simulink model "BMS_EstimateSOC_COM_Harness_MIL"  (R2022b)
settings: configuration reference "BMS_Sw_CodeGenConfig" (kept outside this file)
model workspace: external: MAT-File H:\0\New MAAM\10 - MBD\Battary Management System\SWE.3 CDD\DataTypes\Data_Script.mat (data not in the file)
undefined symbols (not defined in the file): Ion, Lithium
libraries: spsIdealSwitchLib x3, spsBatteryLib x1, spsParallelRLCBranchLib x1, spspowerguiLib x1
settings Model: DataDictionary=BMS_Arch_DD.sldd  Creator=MAAM  LastModifiedBy=MAAM
settings ConfigSetRef: SourceName=BMS_Sw_CodeGenConfig

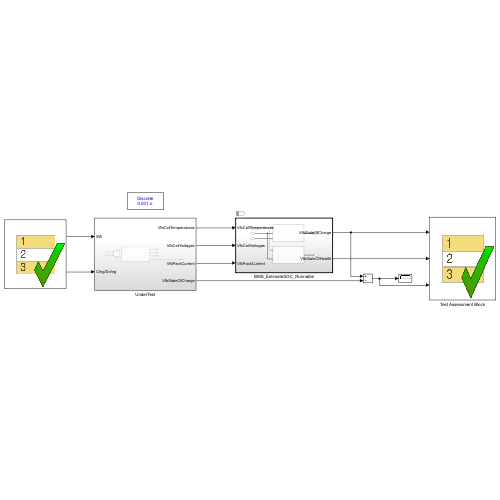
[thumbnail: Simulink's stored preview of the top-level diagram]
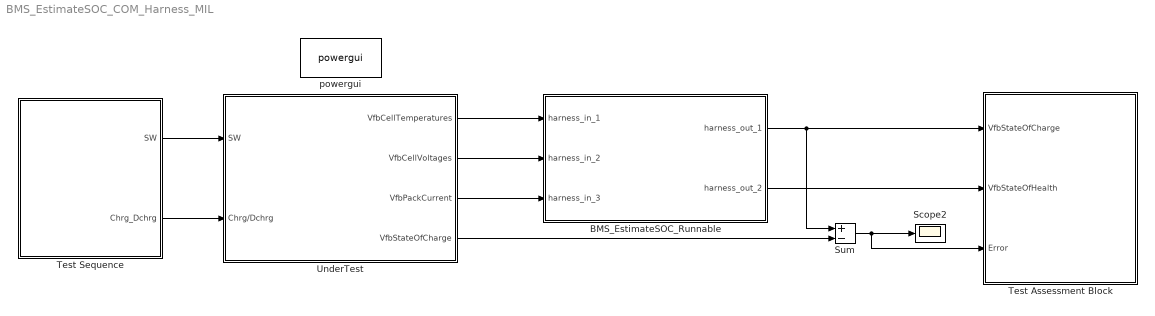
== system BMS_EstimateSOC_COM_Harness_MIL ==
  BMS_EstimateSOC_Runnable : Subsystem  Tag=__SL_testing_harness_stub_  Priority=3
  Scope2 : Scope
  Sum : Sum  Inputs=+-
  Test Assessment Block : Test Sequence  Tag=__SLT_ASMT__  TreatAsAtomicUnit=on
  Test Sequence : Test Sequence  TreatAsAtomicUnit=on
  UnderTest : Subsystem
  powergui : spspowerguiLib/powergui  Priority=1  SimulationMode=Discrete  SampleTime=1e-3  frequency=60  Iterations=50  frequencyindice=0  Pbase=100e6  ErrMax=1e-4  UnitsV=kV  UnitsW=MW  buscounter=0  FunctionMessages=off  echomessages=off  EnableUseOfTLC=off  CurrentSourceSwitches=off  DisableSnubberDevices=off  DisableRonSwitches=off  DisableVfSwitches=off  DisplayEquations=off  AutomaticDiscreteSolvers=off  SolverType=Tustin/Backward Euler (TBE)  Interpol=off  ExternalGateDelay=off  methode=off  Ts=100  x0status=blocks  SPID=on  SwTol=0  HookPort=off  NonlinearTolerance=1e-4  nMaxIteration=100  ContinueOnMaxIteration=off  RestoreLinks=warning  ResistiveCurrentMeasurement=off  Frange=[0:2:500]  Ylog=off  Xlog=on  ShowGrid=off  save=off  variable=ZData  structure=0  ZoomFFT=off  StartTime=0.0  cycles=1  DisplayStyle=1  fundamental=60  FreqAxis=off  MaxFrequency=1000  frequencyindicesteady=1  RmsSteady=1  display=off
  wires:
  BMS_EstimateSOC_Runnable/1(harness_out_1) -> Sum/1, Test Assessment Block/1(VfbStateOfCharge)
  BMS_EstimateSOC_Runnable/2(harness_out_2) -> Test Assessment Block/2(VfbStateOfHealth)
  Sum/1 -> Scope2/1, Test Assessment Block/3(Error)
  Test Sequence/1(SW) -> UnderTest/1(SW)
  Test Sequence/2(Chrg_Dchrg) -> UnderTest/2(Chrg/Dchrg)
  UnderTest/1(VfbCellTemperatures) -> BMS_EstimateSOC_Runnable/1(harness_in_1)
  UnderTest/2(VfbCellVoltages) -> BMS_EstimateSOC_Runnable/2(harness_in_2)
  UnderTest/3(VfbPackCurrent) -> BMS_EstimateSOC_Runnable/3(harness_in_3)
  UnderTest/4(VfbStateOfCharge) -> Sum/2

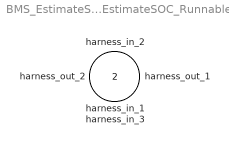
== system BMS_EstimateSOC_COM_Harness_MIL/BMS_EstimateSOC_Runnable ==
  harness_in_1 : Inport
  harness_in_2 : Inport  Port=2
  harness_in_3 : Inport  Port=3
  harness_out_1 : Outport
  harness_out_2 : Outport  Port=2

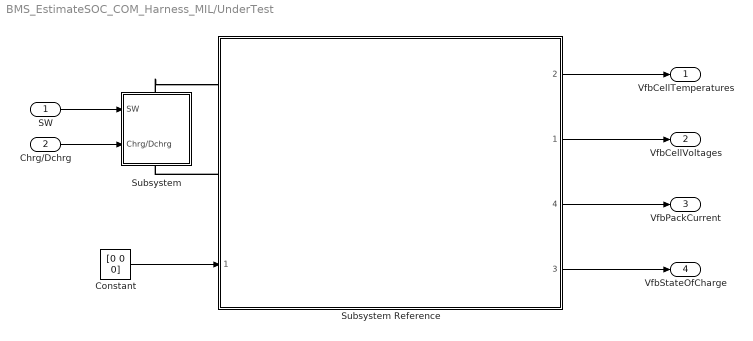
== system BMS_EstimateSOC_COM_Harness_MIL/UnderTest ==
  SW : Inport
  Chrg/Dchrg : Inport  Port=2
  Constant : Constant  Value=[0 0 0]
  Subsystem : Subsystem
      settings: PortSchema="{\"entries\":[{\"content\":{\"sides\":[{\"content\":{\"connectorIds\":[\"LConn1\"]},\"type\":\"ConnectorPlacement.EquallySpacedRectSide\",\"uuid\":\"a461fc5f-bdec-4de1-a769-19a6913359cb\"},{\"content\":{\"connectorIds\":[\"RConn1\"],\"side\":\"RIGHT\"},\"type\":\"ConnectorPlacement.EquallySpacedRectSide\",\"uuid\":\"53dfe770-afde-41f9-b1fd-6523bad3a9ef\"},{\"content\":{\"connectorIds\":[],\"side\":\"TOP\"},\"type\":\"ConnectorPlacement.EquallySpacedRectSide\",\"uuid\":\"157c2878-8b7f-49af-a18e-5ca91668c703\"},{\"content\":{\"connectorIds\":[\"In1\",\"In2\"],\"side\":\"BOTTOM\"},\"type\":\"ConnectorPlacement.EquallySpacedRectSide\",\"uuid\":\"a113e167-ab7e-4584-b97c-54a0a3809f54\"}]},\"type\":\"ConnectorPlacement.EquallySpacedConnector\",\"uuid\":\"fefc71e0-0cbe-4397-b099-f68d58411951\"}],\"packageUris\":[\"http://schema.mathworks.com/mf0/Connector/R2020b\"],\"version\":\"1.0\"}"
  Subsystem Reference : Subsystem  ReferencedSubsystem=Batter_Pack_Sim
      settings: PortSchema="{\"entries\":[{\"content\":{\"sides\":[{\"content\":{\"connectorIds\":[\"LConn1\",\"LConn2\",\"In1\"]},\"type\":\"ConnectorPlacement.EquallySpacedRectSide\",\"uuid\":\"5451cb71-15b5-4b08-b1e3-78543f6c5322\"},{\"content\":{\"connectorIds\":[\"Out2\",\"Out1\",\"Out4\",\"Out3\"],\"side\":\"RIGHT\"},\"type\":\"ConnectorPlacement.EquallySpacedRectSide\",\"uuid\":\"e4bd4e19-96bf-4958-bcea-cb5b9e999de9\"},{\"content\":{\"connectorIds\":[],\"side\":\"TOP\"},\"type\":\"ConnectorPlacement.EquallySpacedRectSide\",\"uuid\":\"ab10f796-18a4-45ff-a38a-380d34cf2a1b\"}]},\"type\":\"ConnectorPlacement.EquallySpacedConnector\",\"uuid\":\"eded12b9-95b7-465b-88e8-d172ae90f9f6\"}],\"packageUris\":[\"http://schema.mathworks.com/mf0/Connector/R2020b\"],\"version\":\"1.0\"}"
  VfbCellTemperatures : Outport
  VfbCellVoltages : Outport  Port=2
  VfbPackCurrent : Outport  Port=3
  VfbStateOfCharge : Outport  Port=4
  wires:
  Subsystem Reference/2 -> VfbCellTemperatures/1
  Subsystem Reference/1 -> VfbCellVoltages/1
  SW/1 -> Subsystem/1(SW)
  Subsystem Reference/3 -> VfbStateOfCharge/1
  Subsystem Reference/4 -> VfbPackCurrent/1
  Chrg/Dchrg/1 -> Subsystem/2(Chrg/Dchrg)
  Constant/1 -> Subsystem Reference/1
  connections:
  Subsystem/LConn1 -- Subsystem Reference/LConn1
  Subsystem Reference/LConn2 -- Subsystem/RConn1

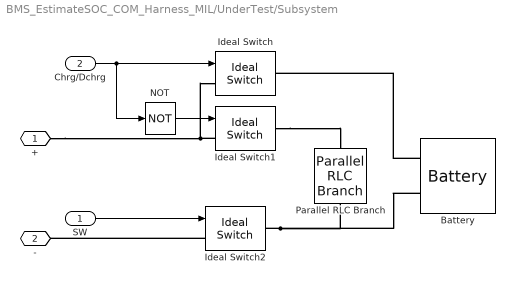
== system BMS_EstimateSOC_COM_Harness_MIL/UnderTest/Subsystem ==
  SW : Inport
  Chrg/Dchrg : Inport  Port=2
  Battery : spsBatteryLib/Battery  BatType=Lithium-Ion  ShowTempParam=off  ThermalPreset=no  ShowAgeParam=off  NomV=3*4.2  NomQ=150  SOC=100  Batt_Tr=1  PresetModel=on  MaxQ=150  MinV=9.45  FullV=14.6662  Dis_rate=65.2174  R=0.00084  Normal_OP=135.6522  expZone="[13.6129      7.36957]"  current=[6.5 13 32.5]  Units=Time  Tci=20  NomT=20  T2=-30  MaxQ2=4.8  FullV2=7.1  Normal_OP2=5.655  expZone2="[6.58           1]"  Rca=0.6  ti=2000  Dp=0  Neq0=0  Tsim=1e6  Ta1=25  Qeol=5.4*0.9  Reol=0.013333*1.2  Char_age=[2.3478, 3]  Dis_age=[2.3478, 10]  N1=1500  N2=10500  N3=1000  N4=1400  Ta2=45  N5=950
  Ideal Switch : spsIdealSwitchLib/Ideal Switch  Ron=0.001  Lon=0  IC=0  Rs=1e5  Cs=inf  Measurements=off
  Ideal Switch1 : spsIdealSwitchLib/Ideal Switch  Ron=0.001  Lon=0  IC=0  Rs=1e5  Cs=inf  Measurements=off
  Ideal Switch2 : spsIdealSwitchLib/Ideal Switch  Ron=0.001  Lon=0  IC=0  Rs=1e5  Cs=inf  Measurements=off
  NOT : Logic  Operator=NOT  IconShape=distinctive  AllPortsSameDT=off  OutDataTypeStr=boolean
  Parallel RLC Branch : spsParallelRLCBranchLib/Parallel RLC Branch  LConnTagsString=a  RConnTagsString=__new0  BranchType=R  Resistance=1  Inductance=1e-3  SetiL0=off  InitialCurrent=0  Capacitance=1e-6  Setx0=off  InitialVoltage=0  Measurements=None
  + : PMIOPort  Side=Left
  - : PMIOPort  Port=2  Side=Right
  wires:
  SW/1 -> Ideal Switch2/1
  NOT/1 -> Ideal Switch1/1
  Chrg/Dchrg/1 -> Ideal Switch/1, NOT/1
  connections:
  Ideal Switch2/LConn1 -- -/RConn1
  Ideal Switch2/RConn1 -- Parallel RLC Branch/RConn1 -- Battery/LConn2
  Ideal Switch1/RConn1 -- Parallel RLC Branch/LConn1
  +/RConn1 -- Ideal Switch/LConn1 -- Ideal Switch1/LConn1
  Battery/LConn1 -- Ideal Switch/RConn1

== stateflow chart BMS_EstimateSOC_COM_Harness_MIL/Test Assessment Block ==
  state Run
    state step_1_1
    state step_1_2
    (default) -> (junction 22)
    Run -> (junction 22)
    (junction 22) -> (junction 23) [order 1] : [t < 5
        | ]
    (junction 23) -> step_1_1 [order 1] : [~in(Run.step_1_1)]
    (junction 23) -> (junction 26) [order 2]
    (junction 31) -> (junction 32)
    (junction 32) -> step_1_2 [order 1] : [~in(Run.step_1_2)]
    (junction 32) -> (junction 35) [order 2]
    (junction 22) -> (junction 31) [order 2]
  (default) -> Run
  data: VfbStateOfCharge input single size=[3]; VfbStateOfHealth input single size=[3]; Error input

== stateflow chart BMS_EstimateSOC_COM_Harness_MIL/Test Sequence ==
  settings: updateMethod=DISCRETE  sampleTime=0.2
  state Cold_Start
    state Run
      SW = 1;
      Chrg_Dchrg = 0;
    state step_1
      SW = 0;
      Chrg_Dchrg = 0;
    state step_2
    (default) -> Cold_Start.Run
    Cold_Start.Run -> Cold_Start.step_1 : [
        | after(100, sec)
        | ]
    Cold_Start.step_1 -> Cold_Start.Run : [
        | after(100, sec)
        | ]
  state High_Puls_Discharge
    state Run
      SW = 1;
      Chrg_Dchrg = 0;
    state step_1
      SW = 0;
      Chrg_Dchrg = 0;
    state step_2
    (default) -> High_Puls_Discharge.Run
    High_Puls_Discharge.Run -> High_Puls_Discharge.step_1 : [
        | after(100, sec)
        | ]
    High_Puls_Discharge.step_1 -> High_Puls_Discharge.Run : [
        | after(100, sec)
        | ]
  state Regenerative_Braking
    state Run
      SW = 1;
      Chrg_Dchrg = 0;
    state step_1
      SW = 0;
      Chrg_Dchrg = 0;
    state step_2
    (default) -> Regenerative_Braking.Run
    Regenerative_Braking.Run -> Regenerative_Braking.step_1 : [
        | after(100, sec)
        | ]
    Regenerative_Braking.step_1 -> Regenerative_Braking.Run : [
        | after(100, sec)
        | ]
  state Idle_Rest
    state Run
      SW = 1;
      Chrg_Dchrg = 0;
    state step_1
      SW = 0;
      Chrg_Dchrg = 0;
    state step_2
    (default) -> Idle_Rest.Run
    Idle_Rest.Run -> Idle_Rest.step_1 : [
        | after(100, sec)
        | ]
    Idle_Rest.step_1 -> Idle_Rest.Run : [
        | after(100, sec)
        | ]
  state Dynamic_Test
    state Run
      SW = 1;
      Chrg_Dchrg = 0;
    state step_1
      SW = 0;
      Chrg_Dchrg = 0;
    state step_2
    (default) -> Dynamic_Test.Run
    Dynamic_Test.Run -> Dynamic_Test.step_1 : [
        | after(100, sec)
        | ]
    Dynamic_Test.step_1 -> Dynamic_Test.Run : [
        | after(100, sec)
        | ]
  (default) -> Cold_Start [order 1] : [Active_Scenario_Index == 1]
  (default) -> High_Puls_Discharge [order 2] : [Active_Scenario_Index == 2]
  (default) -> Regenerative_Braking [order 3] : [Active_Scenario_Index == 3]
  (default) -> Idle_Rest [order 4] : [Active_Scenario_Index == 4]
  (default) -> Dynamic_Test [order 5] : {assert(Active_Scenario_Index == 5,'The value of Scenario Parameter ''Active_Scenario_Index'' is not valid. Use the index of the scenario to specify it.')}
  data: SW output single size=1; Chrg_Dchrg output single size=1; Active_Scenario_Index parameter =1
